simulink model "AirbrakeFlightSim_R2022a"  (R2022a)
settings: Solver=VariableStepAuto  StartTime=0.0  StopTime=18  RelTol=1e-3  AbsTol=1e-6
model workspace (MAT data in the model file):
  test = 1
undefined symbols (not defined in the file or in its folder): accelerometer, atm, gyroscope, model_g_mps2, true_g_mps2, wn, zeta
libraries: simulink x14, simulink_extras x3, aerolibnav x3, matrix_library x2, slpidlib x1
(part 2 of 2)

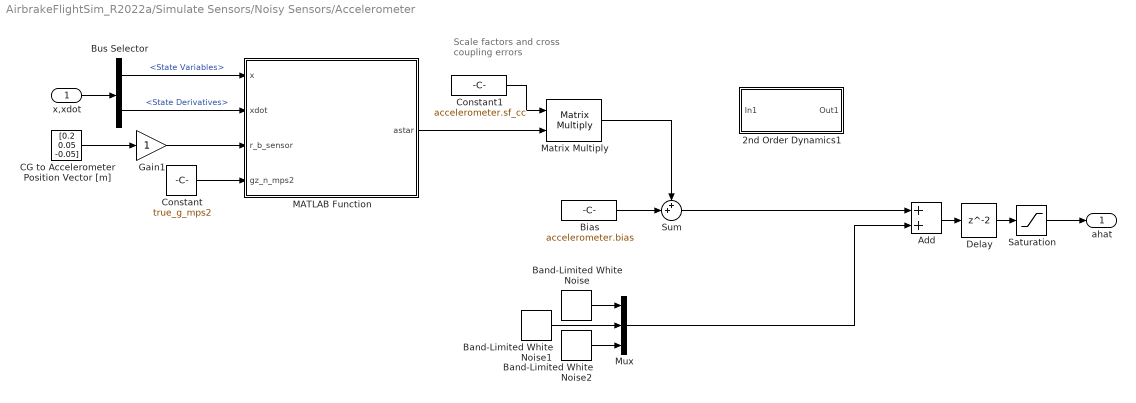
== system AirbrakeFlightSim_R2022a/Simulate Sensors/Noisy Sensors/Accelerometer ==
  note: Scale factors and
      | cross coupling errors
  x,xdot : Inport
  2nd Order Dynamics1 : Subsystem
  Add : Sum
  Band-Limited White Noise : simulink/Sources/Band-Limited White Noise  Cov=[1e-3]  Ts=1/100  seed=[23341]
  Band-Limited White Noise1 : simulink/Sources/Band-Limited White Noise  Cov=[1e-3]  Ts=1/100  seed=[23341]
  Band-Limited White Noise2 : simulink/Sources/Band-Limited White Noise  Cov=[1e-3]  Ts=1/100  seed=[23341]
  Bias : Constant  Value=accelerometer.bias
  Bus Selector : BusSelector  OutputSignals=State Variables,State Derivatives
  CG to Accelerometer Position Vector [m] : Constant  Value=[0.2 0.05 -0.05]
  Constant : Constant  Value=true_g_mps2
  Constant1 : Constant  Value=accelerometer.sf_cc
  Delay : Delay  SampleTime=1/100
  Gain1 : Gain
  MATLAB Function : MATLAB Function  TreatAsAtomicUnit=on
  Matrix Multiply : Product  Multiplication=Matrix(*)
  Mux : Mux  Inputs=3
  Saturation : Saturate  UpperLimit=16*9.81  LowerLimit=-16*9.81
  Sum : Sum  Inputs=++|
  ahat : Outport
  wires:
  Delay/1 -> Saturation/1
  Band-Limited White Noise1/1 -> Mux/2
  Band-Limited White Noise2/1 -> Mux/3
  Band-Limited White Noise/1 -> Mux/1
  Add/1 -> Delay/1
  Saturation/1 -> ahat/1
  x,xdot/1 -> Bus Selector/1
  Bus Selector/1 -> MATLAB Function/1(x)  "<State Variables>"
  Bus Selector/2 -> MATLAB Function/2(xdot)  "<State Derivatives>"
  CG to Accelerometer Position Vector [m]/1 -> Gain1/1
  Constant/1 -> MATLAB Function/4(gz_n_mps2)
  Mux/1 -> Add/2
  Gain1/1 -> MATLAB Function/3(r_b_sensor)
  MATLAB Function/1(astar) -> Matrix Multiply/2
  Constant1/1 -> Matrix Multiply/1
  Sum/1 -> Add/1
  Matrix Multiply/1 -> Sum/1
  Bias/1 -> Sum/2

== system AirbrakeFlightSim_R2022a/Simulate Sensors/Noisy Sensors/Altimeter ==
  x,xdot : Inport
  Add : Sum
  Band-Limited White Noise : simulink/Sources/Band-Limited White Noise  Cov=[0.01]  Ts=1/25  seed=[23341]
  Bus Selector : BusSelector  OutputSignals=State Variables
  Delay1 : Delay  SampleTime=1/25
  Gain : Gain  Gain=-1
  Saturation : Saturate  UpperLimit=20000  LowerLimit=-20000
  Scope : Scope
  Selector : Selector  InputPortWidth=12  IndexOptions=Index vector (dialog)  Indices=[12]  OutputSizes=1
  altitudehat : Outport
  wires:
  Saturation/1 -> altitudehat/1
  Add/1 -> Delay1/1
  Delay1/1 -> Saturation/1
  Selector/1 -> Gain/1  "p_down_m"
  Gain/1 -> Add/1  "altitude"
  x,xdot/1 -> Bus Selector/1
  Bus Selector/1 -> Selector/1  "<State Variables>"
  Band-Limited White Noise/1 -> Add/2

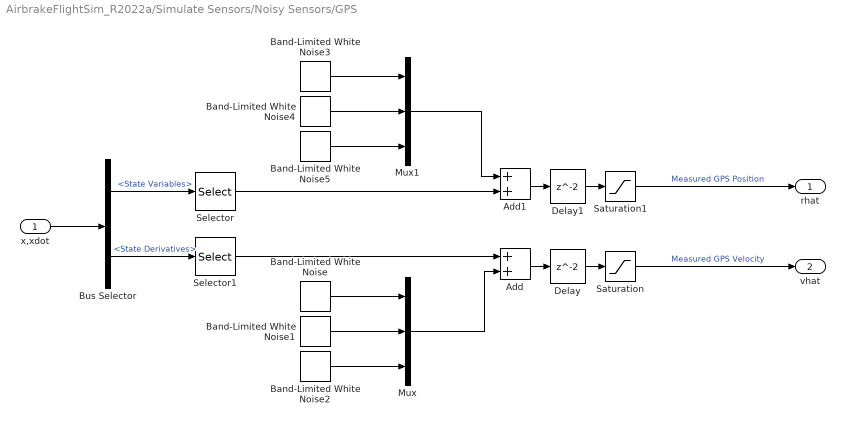
== system AirbrakeFlightSim_R2022a/Simulate Sensors/Noisy Sensors/GPS ==
  x,xdot : Inport
  Add : Sum
  Add1 : Sum
  Band-Limited White Noise{,1..5} (6 alike) : simulink/Sources/Band-Limited White Noise  Cov=[1e-3*pi/180]  Ts=1/100  seed=[23341]
  Bus Selector : BusSelector  OutputSignals=State Variables,State Derivatives
  Delay : Delay  SampleTime=1/100
  Delay1 : Delay  SampleTime=1/100
  Mux : Mux  Inputs=3
  Mux1 : Mux  Inputs=3
  Saturation : Saturate  UpperLimit=500*pi/180  LowerLimit=-500*pi/180
  Saturation1 : Saturate  UpperLimit=500*pi/180  LowerLimit=-500*pi/180
  Selector : Selector  InputPortWidth=12  IndexOptions=Index vector (dialog)  Indices=[10 11 12]  OutputSizes=1
  Selector1 : Selector  InputPortWidth=12  IndexOptions=Index vector (dialog)  Indices=[10 11 12]  OutputSizes=1
  rhat : Outport
  vhat : Outport  Port=2
  wires:
  Delay/1 -> Saturation/1
  Band-Limited White Noise1/1 -> Mux/2
  Band-Limited White Noise2/1 -> Mux/3
  Band-Limited White Noise/1 -> Mux/1
  Add/1 -> Delay/1
  x,xdot/1 -> Bus Selector/1
  Mux/1 -> Add/2
  Bus Selector/1 -> Selector/1  "<State Variables>"
  Bus Selector/2 -> Selector1/1  "<State Derivatives>"
  Band-Limited White Noise5/1 -> Mux1/3
  Band-Limited White Noise4/1 -> Mux1/2
  Band-Limited White Noise3/1 -> Mux1/1
  Selector1/1 -> Add/1
  Add1/1 -> Delay1/1
  Delay1/1 -> Saturation1/1
  Mux1/1 -> Add1/1
  Selector/1 -> Add1/2
  Saturation/1 -> vhat/1  "Measured GPS Velocity"
  Saturation1/1 -> rhat/1  "Measured GPS Position"

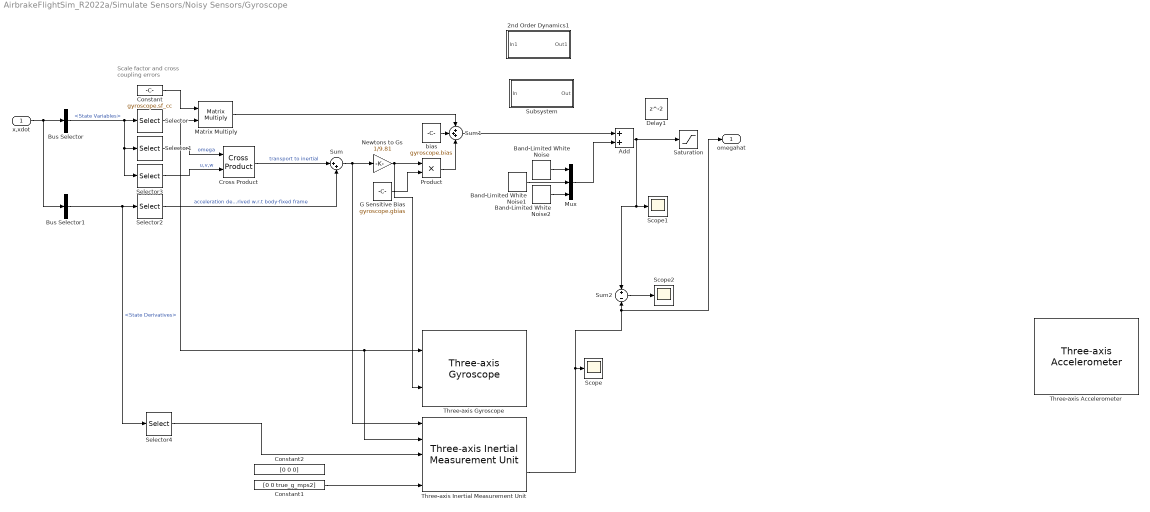
== system AirbrakeFlightSim_R2022a/Simulate Sensors/Noisy Sensors/Gyroscope ==
  note: Scale factor and
      | cross coupling errors
  x,xdot : Inport
  2nd Order Dynamics1 : Subsystem
  Add : Sum
  Band-Limited White Noise : simulink/Sources/Band-Limited White Noise  Cov=[1e-3]  Ts=1/10  seed=23093
  Band-Limited White Noise1 : simulink/Sources/Band-Limited White Noise  Cov=[1e-3]  Ts=1/10  seed=23094
  Band-Limited White Noise2 : simulink/Sources/Band-Limited White Noise  Cov=[1e-3]  Ts=1/10  seed=23095
  Bus Selector : BusSelector  OutputSignals=State Variables
  Bus Selector1 : BusSelector  OutputSignals=State Derivatives
  Constant : Constant  Value=gyroscope.sf_cc
  Constant1 : Constant  Value=[0 0 true_g_mps2]
  Constant2 : Constant  Value=[0 0 0]
  Cross Product : matrix_library/Cross Product
      settings: SourceProductBaseCode=SL
  Delay1 : Delay  SampleTime=1/100
  G Sensitive Bias : Constant  Value=gyroscope.gbias
  Matrix Multiply : Product  Multiplication=Matrix(*)
  Mux : Mux  Inputs=3
  Newtons to Gs : Gain  Gain=1/9.81
  Product : Product
  Saturation : Saturate  UpperLimit=500*pi/180  LowerLimit=-500*pi/180
  Scope : Scope
  Scope1 : Scope
  Scope2 : Scope
  Selector : Selector  InputPortWidth=12  IndexOptions=Index vector (dialog)  Indices=[4 5 6]  OutputSizes=1
  Selector1 : Selector  InputPortWidth=12  IndexOptions=Index vector (dialog)  Indices=[4 5 6]  OutputSizes=1
  Selector2 : Selector  InputPortWidth=12  IndexOptions=Index vector (dialog)  Indices=[1 2 3]  OutputSizes=1
  Selector3 : Selector  InputPortWidth=12  IndexOptions=Index vector (dialog)  Indices=[1 2 3]  OutputSizes=1
  Selector4 : Selector  InputPortWidth=12  IndexOptions=Index vector (dialog)  Indices=[4 5 6]  OutputSizes=1
  Subsystem : Subsystem
  Sum : Sum  Inputs=|++
  Sum1 : Sum  Inputs=+++
  Sum2 : Sum  Inputs=+|-
  Three-axis Accelerometer : aerolibnav/Three-axis Accelerometer  units=Metric (MKS)  acc=[0 0 0]  gtype=on  dtype_a=on  w_a=190  z_a=0.707  a_sf_cc=[1 0 0; 0 1 0; 0 0 1]  a_bias=[0 0 0]  a_Ts=0  a_rand=on  a_seeds=[23093 23094 23095]  a_pow=[0.001 0.001 0.001]  a_sat="[-inf  -inf  -inf  inf inf inf]"
      settings: SourceProductBaseCode=AE
  Three-axis Gyroscope : aerolibnav/Three-axis Gyroscope  dtype_g=on  w_g=wn  z_g=zeta  g_sf_cc=gyroscope.sf_cc  g_bias=gyroscope.bias  g_sen=gyroscope.gbias  g_Ts=1/100  g_rand=on  g_seeds=[23093 23094 23095]  g_pow=[0.001 0.001 0.001]  g_sat="[-inf  -inf  -inf  inf inf inf]"
      settings: SourceProductBaseCode=AE
  Three-axis Inertial Measurement Unit : aerolibnav/Three-axis Inertial Measurement Unit  units=Metric (MKS)  imu=[0 0 0]  i_Ts=0  dtype_a=off  w_a=wn  z_a=zeta  a_sf_cc=[1 0 0; 0 1 0; 0 0 1]  a_bias=[0 0 0]  a_sat="[-inf  -inf  -inf  inf inf inf]"  dtype_g=off  w_g=wn  z_g=zeta  g_sf_cc=[1 0 0; 0 1 0; 0 0 1]  g_bias=[0 0 0]  g_sens=[0 0 0]  g_sat="[-inf  -inf  -inf  inf inf inf]"  i_rand=on  i_seeds=[23093 23094 23095 23093 23094 23095]  i_pow=[0.001 0.001 0.001 0.001 0.001 0.001]
  bias : Constant  Value=gyroscope.bias
  omegahat : Outport
  wires:
  Add/1 -> Saturation/1, Sum2/1, Scope1/1
  Band-Limited White Noise1/1 -> Mux/2
  Band-Limited White Noise2/1 -> Mux/3
  Band-Limited White Noise/1 -> Mux/1
  x,xdot/1 -> Bus Selector1/1, Bus Selector/1
  Bus Selector/1 -> Selector/1, Selector3/1, Selector1/1  "<State Variables>"
  Mux/1 -> Add/2
  Selector/1 -> Three-axis Gyroscope/1, Three-axis Inertial Measurement Unit/2, Matrix Multiply/2
  Constant/1 -> Matrix Multiply/1
  Bus Selector1/1 -> Selector4/1, Selector2/1  "<State Derivatives>"
  Selector3/1 -> Cross Product/2  "u,v,w"
  Selector1/1 -> Cross Product/1  "omega"
  Cross Product/1 -> Sum/1  "transport to inertial"
  Selector2/1 -> Sum/2  "acceleration derived w.r.t body-fixed frame"
  Sum/1 -> Newtons to Gs/1, Three-axis Inertial Measurement Unit/1
  Newtons to Gs/1 -> Product/1, Three-axis Gyroscope/2
  G Sensitive Bias/1 -> Product/2
  Product/1 -> Sum1/3
  Matrix Multiply/1 -> Sum1/1
  bias/1 -> Sum1/2
  Three-axis Inertial Measurement Unit/2 -> omegahat/1, Sum2/2, Scope/1
  Sum2/1 -> Scope2/1
  Selector4/1 -> Three-axis Inertial Measurement Unit/3
  Constant1/1 -> Three-axis Inertial Measurement Unit/5
  Sum1/1 -> Add/1

== system AirbrakeFlightSim_R2022a/Simulate Sensors/Noisy Sensors/Magnetometer ==
  x,xdot : Inport
  Add : Sum
  Band-Limited White Noise : simulink/Sources/Band-Limited White Noise  Cov=[0.01]  Ts=1/25  seed=[23341]
  Bus Selector : BusSelector  OutputSignals=State Variables
  Delay1 : Delay  SampleTime=1/25
  Saturation : Saturate  UpperLimit=20000  LowerLimit=-20000
  Selector : Selector  InputPortWidth=12  IndexOptions=Index vector (dialog)  Indices=[9]  OutputSizes=1
  headinghat : Outport
  wires:
  Saturation/1 -> headinghat/1
  Add/1 -> Delay1/1
  Delay1/1 -> Saturation/1
  Selector/1 -> Add/1  "yaw"
  x,xdot/1 -> Bus Selector/1
  Bus Selector/1 -> Selector/1  "<State Variables>"
  Band-Limited White Noise/1 -> Add/2

== system AirbrakeFlightSim_R2022a/Simulate True Dynamics 6DOF/Compute Aerodynamic Forces/Angle of Attack ==
  In1 : Inport
  Atan2 : Trigonometry  Operator=atan2
  Demux : Demux  Outputs=3
  alpha : Outport
  wires:
  In1/1 -> Demux/1
  Atan2/1 -> alpha/1
  Demux/3 -> Atan2/1
  Demux/1 -> Atan2/2

== system AirbrakeFlightSim_R2022a/Simulate True Dynamics 6DOF/Compute Aerodynamic Forces/Angle of Sideslip ==
  v : Inport
  V : Inport  Port=2
  Abs : Abs  SaturateOnIntegerOverflow=off
  Asin : Trigonometry  Operator=asin
  Constant : Constant  Value=0
  Divide : Product  Inputs=*/
  Selector : Selector  InputPortWidth=3  IndexOptions=Index vector (dialog)  Indices=[2]  OutputSizes=1
  Switch : Switch  Criteria=u2 > Threshold  SaturateOnIntegerOverflow=off  InputSameDT=off
  beta : Outport
  wires:
  V/1 -> Divide/2
  Divide/1 -> Asin/1
  Asin/1 -> Switch/1, Abs/1
  Switch/1 -> beta/1
  Abs/1 -> Switch/2
  Constant/1 -> Switch/3
  v/1 -> Selector/1
  Selector/1 -> Divide/1

== system AirbrakeFlightSim_R2022a/Simulate True Dynamics 6DOF/Compute Aerodynamic Forces/Dynamic Pressure ==
  V : Inport
  rho : Inport  Port=2
  Constant : Constant  Value=0.5
  Product : Product  Inputs=4
  qbar : Outport
  wires:
  V/1 -> Product/3, Product/2
  rho/1 -> Product/4
  Constant/1 -> Product/1
  Product/1 -> qbar/1

== system AirbrakeFlightSim_R2022a/Simulate True Dynamics 6DOF/Compute Aerodynamic Forces/Mach Number ==
  V : Inport
  c : Inport  Port=2
  Divide : Product  Inputs=*/
  M : Outport
  wires:
  V/1 -> Divide/1
  c/1 -> Divide/2
  Divide/1 -> M/1

== system AirbrakeFlightSim_R2022a/Simulate True Dynamics 6DOF/Compute Aerodynamic Forces/Speed of Sound ==
  Temperature : Inport
  Ratio of specific heats : Gain  Gain=1.4
  Specific gas constant : Gain  Gain=287.05
  Sqrt : Sqrt
  c : Outport
  wires:
  Temperature/1 -> Ratio of specific heats/1
  Ratio of specific heats/1 -> Specific gas constant/1
  Specific gas constant/1 -> Sqrt/1
  Sqrt/1 -> c/1

== system AirbrakeFlightSim_R2022a/Simulate True Dynamics 6DOF/Interpolate Thrust & Mass/Check Motor Burnout ==
  In1 : Inport
  Bus Selector : BusSelector  OutputSignals=Vehicle Properties.Motor Time Breakpoints,Simulation Time
  Gain : Gain  Gain=-1
  checkMotorBurnout : Subsystem
  tag scope: Time_Since_Burnout=global
  wires:
  checkMotorBurnout/1(Time Since Burnout) -> [Time_Since_Burnout]
  In1/1 -> Bus Selector/1
  Bus Selector/1 -> Gain/1  "<Motor Time Breakpoints>"
  Bus Selector/2 -> checkMotorBurnout/2(In2)  "<Simulation Time>"
  Gain/1 -> checkMotorBurnout/1(In1)

== system AirbrakeFlightSim_R2022a/Simulate True Dynamics 6DOF/Interpolate Thrust & Mass/Inertia (UNFINISHED) ==
  In1 : Inport
  Bus Selector : BusSelector  OutputSignals=Vehicle Properties.Vehicle Inertia [kg-m2]
  Out1 : Outport
  wires:
  In1/1 -> Bus Selector/1
  Bus Selector/1 -> Out1/1  "<Vehicle Inertia [kg-m2]>"

== system AirbrakeFlightSim_R2022a/Simulate True Dynamics 6DOF/Interpolate Thrust & Mass/Interpolate Mass ==
  1 : Inport
  Add : Sum
  Bus Selector : BusSelector  OutputSignals=Vehicle Properties.Vehicle Mass [kg],Simulation Time,Vehicle Properties.Motor Mass Breakpoints,Vehicle Properties.Motor Time Breakpoints
  Mass Curve : Lookup_n-D  NumberOfTableDimensions=1  BreakpointsForDimension1Source=Input port  BreakpointsForDimension1=|  TableSource=Input port  Table=|  ExtrapMethod=Clip  UseLastTableValue=on  InternalRulePriority=Speed  RndMeth=Simplest
      BreakpointsForDimension1=|
      | [   2.0000e-02
      |    4.0000e-02
      |    5.5000e-02
      |    7.3000e-02
      |    1.5600e-01
      |    3.9700e-01
      |    6.9100e-01
      |    9.8200e-01
      |    1.4100e+00
      |    1.6960e+00
      |    1.9350e+00
      |    2.0600e+00
      |    2.1030e+00
      |    2.1160e+00
      |    2.1330e+00
      |    2.1630e+00
      |    2.2140e+00
      |    2.2440e+00
      |    2.2960e+00
      |    2.3090e+00]
      Table=|
      | [4.8137e+01
      |    2.1073e+03
      |    2.2892e+03
      |    2.1501e+03
      |    2.1020e+03
      |    2.1501e+03
      |    2.1555e+03
      |    2.1180e+03
      |    2.0004e+03
      |    1.8987e+03
      |    1.8399e+03
      |    1.8185e+03
      |    1.6527e+03
      |    1.3746e+03
      |    9.3600e+02
      |    5.3486e+02
      |    2.4069e+02
      |    1.1232e+02
      |    5.3490e+00
      |             0]
      settings: InputPortMap=u0,p221,p5
  Mass : Outport
  wires:
  Mass Curve/1 -> Add/2
  Add/1 -> Mass/1
  1/1 -> Bus Selector/1
  Bus Selector/2 -> Mass Curve/1  "<Simulation Time>"
  Bus Selector/3 -> Mass Curve/2  "<Motor Mass Breakpoints>"
  Bus Selector/4 -> Mass Curve/3  "<Motor Time Breakpoints>"
  Bus Selector/1 -> Add/1  "<Vehicle Mass [kg]>"

== system AirbrakeFlightSim_R2022a/Simulate True Dynamics 6DOF/Interpolate Thrust & Mass/Interpolate Thrust ==
  In1 : Inport
  Bus Selector : BusSelector  OutputSignals=Motor Thrust Breakpoints,Motor Time Breakpoints
  Bus Selector1 : BusSelector  OutputSignals=Simulation Time,Vehicle Properties
  "Thrust Curve " : Lookup_n-D  NumberOfTableDimensions=1  BreakpointsForDimension1Source=Input port  BreakpointsForDimension1=|  TableSource=Input port  Table=|  ExtrapMethod=Clip  InternalRulePriority=Speed  RndMeth=Simplest
      BreakpointsForDimension1=|
      | [   2.0000e-02
      |    4.0000e-02
      |    5.5000e-02
      |    7.3000e-02
      |    1.5600e-01
      |    3.9700e-01
      |    6.9100e-01
      |    9.8200e-01
      |    1.4100e+00
      |    1.6960e+00
      |    1.9350e+00
      |    2.0600e+00
      |    2.1030e+00
      |    2.1160e+00
      |    2.1330e+00
      |    2.1630e+00
      |    2.2140e+00
      |    2.2440e+00
      |    2.2960e+00
      |    2.3090e+00]
      Table=|
      | [4.8137e+01
      |    2.1073e+03
      |    2.2892e+03
      |    2.1501e+03
      |    2.1020e+03
      |    2.1501e+03
      |    2.1555e+03
      |    2.1180e+03
      |    2.0004e+03
      |    1.8987e+03
      |    1.8399e+03
      |    1.8185e+03
      |    1.6527e+03
      |    1.3746e+03
      |    9.3600e+02
      |    5.3486e+02
      |    2.4069e+02
      |    1.1232e+02
      |    5.3490e+00
      |             0]
      settings: InputPortMap=u0,p221,p5
  Out1 : Outport
  wires:
  "Thrust Curve "/1 -> Out1/1
  Bus Selector/2 -> "Thrust Curve "/3  "<Motor Time Breakpoints>"
  Bus Selector/1 -> "Thrust Curve "/2  "<Motor Thrust Breakpoints>"
  Bus Selector1/1 -> "Thrust Curve "/1  "<Simulation Time>"
  In1/1 -> Bus Selector1/1
  Bus Selector1/2 -> Bus Selector/1  "<Vehicle Properties>"

== system AirbrakeFlightSim_R2022a/Simulate Sensors/Noisy Sensors/Accelerometer/2nd Order Dynamics1 ==
  In1 : Inport
  Gain : Gain  Gain=wn*wn
  Gain1 : Gain  Gain=2*zeta*wn
  "Integrator, Second-Order" : SecondOrderIntegrator
  Sum : Sum  Inputs=|++
  Sum1 : Sum  Inputs=|++
  Out1 : Outport
  wires:
  In1/1 -> Sum/1
  Sum/1 -> Gain/1
  Gain/1 -> Sum1/1
  Sum1/1 -> "Integrator, Second-Order"/1
  "Integrator, Second-Order"/1 -> Sum/2, Out1/1
  "Integrator, Second-Order"/2 -> Gain1/1
  Gain1/1 -> Sum1/2

== system AirbrakeFlightSim_R2022a/Simulate Sensors/Noisy Sensors/Gyroscope/2nd Order Dynamics1 ==
  In1 : Inport
  Gain : Gain  Gain=wn*wn
  Gain1 : Gain  Gain=2*zeta*wn
  "Integrator, Second-Order" : SecondOrderIntegrator
  Sum : Sum  Inputs=|+-
  Sum1 : Sum  Inputs=|+-
  Out1 : Outport
  wires:
  In1/1 -> Sum/1
  Sum/1 -> Gain/1
  Gain/1 -> Sum1/1
  Sum1/1 -> "Integrator, Second-Order"/1
  "Integrator, Second-Order"/1 -> Sum/2, Out1/1
  "Integrator, Second-Order"/2 -> Gain1/1
  Gain1/1 -> Sum1/2

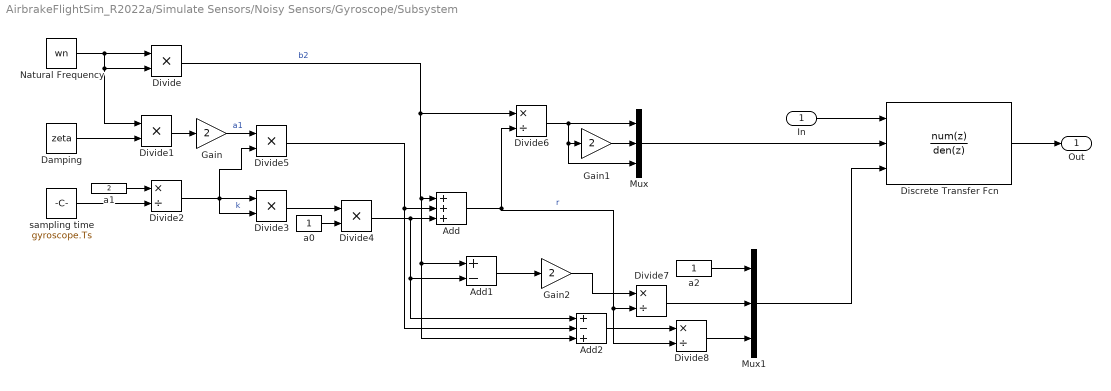
== system AirbrakeFlightSim_R2022a/Simulate Sensors/Noisy Sensors/Gyroscope/Subsystem ==
  In : Inport
  Add : Sum  Inputs=+++
  Add1 : Sum  Inputs=+-
  Add2 : Sum  Inputs=+-+
  Damping : Constant  Value=zeta
  Discrete Transfer Fcn : DiscreteTransferFcn  NumeratorSource=Input port  DenominatorSource=Input port  SampleTime=gyroscope.Ts  a0EqualsOne=on
      settings: InputPortMap=u0,p1,p3
  Divide{,1,3..5} (5 alike) : Product  Inputs=**
  Divide{2,6..8} (4 alike) : Product  Inputs=*/
  Gain : Gain  Gain=2
  Gain1 : Gain  Gain=2
  Gain2 : Gain  Gain=2
  Mux : Mux  Inputs=3
  Mux1 : Mux  Inputs=3
  Natural Frequency : Constant  Value=wn
  a0 : Constant
  a1 : Constant  Value=2
  a2 : Constant
  sampling time : Constant  Value=gyroscope.Ts
  Out : Outport  VectorParamsAs1DForOutWhenUnconnected=off
  wires:
  Divide1/1 -> Gain/1
  Divide8/1 -> Mux1/3
  Divide7/1 -> Mux1/2
  Divide2/1 -> Divide5/2, Divide3/2, Divide3/1  "k"
  Add/1 -> Divide8/2, Divide7/2, Divide6/2  "r"
  In/1 -> Discrete Transfer Fcn/1
  Gain/1 -> Divide5/1  "a1"
  Mux1/1 -> Discrete Transfer Fcn/3
  Add1/1 -> Gain2/1
  Mux/1 -> Discrete Transfer Fcn/2
  Gain1/1 -> Mux/2
  Divide5/1 -> Add2/2, Add/2
  Gain2/1 -> Divide7/1
  Add2/1 -> Divide8/1
  sampling time/1 -> Divide2/2
  a1/1 -> Divide2/1
  Divide3/1 -> Divide4/1
  Divide4/1 -> Add2/1, Add1/2, Add/3
  a2/1 -> Mux1/1
  Divide/1 -> Divide6/1, Add2/3, Add1/1, Add/1  "b2"
  a0/1 -> Divide4/2
  Damping/1 -> Divide1/2
  Discrete Transfer Fcn/1 -> Out/1
  Natural Frequency/1 -> Divide/1, Divide/2, Divide1/1
  Divide6/1 -> Mux/3, Gain1/1, Mux/1

== system AirbrakeFlightSim_R2022a/Simulate True Dynamics 6DOF/Interpolate Thrust & Mass/Check Motor Burnout/checkMotorBurnout ==
  In1 : Inport
  In2 : Inport  Port=2
  Add : Sum
  Selector : Selector  InputPortWidth=20  IndexOptions=Index vector (dialog)  Indices=[20]  OutputSizes=1
  Time Since Burnout : Outport
  wires:
  Selector/1 -> Add/1
  Add/1 -> Time Since Burnout/1
  In2/1 -> Add/2
  In1/1 -> Selector/1

== matlab function AirbrakeFlightSim_R2022a/Simulate True Dynamics 6DOF/Compute Aerodynamic Forces/MATLAB Function ==
  data: drag_characteristics input; fins input; velocity_vec input; D output; alpha_rad input; beta_rad input; qbar_kgpms2 input; mach input; Y output; L output
function [D,Y,L] = compute_aerodynamic_forces(drag_characteristics,fins, velocity_vec, alpha_rad,beta_rad,qbar_kgpms2, mach)
% aero_w_N = rocketAeroModel(alpha_rad, beta_rad, qbar_kgpms2, vehicle)
% 
% Computes the aerodynamic force vector of launch vehicle with fins placed
% symmetrically about the longitudinal axis. The body-fixed frame must
% have the y-axis along any fin.
% 
% Inputs:
%   drag_characteristics - vehicle CD*S   
%
%   fins - vector containing vehicle parameters
%       fins.num_fins - number of fins
%       fins.CL_alpha - slope of the lift coeff vs angle of attack curve
%       fins.planform_area - exposed planform area of fin
%
%   velocity_vec - 3x1 vector containing u,v,w body-fixed inertial velocities
%
%   alpha_rad - vehicle angle of attack in radians
%
%   beta_rad - vehicle angle of sideslip in radians
%
%   qbar_kgpms2 - vehicle dynamic pressure in Newtons per meter squared
%
%   mach - mach number
%
% Outputs:
%   aero_B_N - aerodynamic force vector resolved in Body-Fixed coordinates
%   and expressed in Newtons.
%       3 x 1 vector

%% Old Attempt
% % Extract vehicle properties
% CL_alpha = vehicle.fins.CL_alpha;
% CD = vehicle.cd;
% vehicle_area = vehicle.area;
% 
% % Compute drag (fixed Cd does not vary with AoA)
% D = CD*qbar_kgpms2*vehicle_area;
% 
% % Compute lift coeff
% CL = CL_alpha * alpha_rad;
% L = CL*qbar_kgpms2*vehicle_area;
% 
% aero_w_N = [D 0 L];

%% New attempt

% Define vehicle parameters
C_N_alpha_fins = fins(1);
fin_area = fins(2);
num_fins = fins(3);
C_N_alpha_nosecone = 2;


% Initialize aerodynamic force vector resolved in wind axes
aero_w_N = [0 0 0]';

% Fins
for ii = 0:num_fins-1
    
    % Fin position along body diameter
    psi = (2*pi/num_fins)*ii;

    % angle of attack relative to i'th fin
    alpha_i = alpha_rad*cos(psi) - beta_rad*sin(psi);

    % Magnitude of normal force from i'th fin
    N = qbar_kgpms2 * fin_area * C_N_alpha_fins * alpha_i;

    % Direction of normal force
    n_hat = [0 -sin(psi) cos(psi)]';

    % Normal force vector for i'th fin
    F_i = N*n_hat;
    
    % Add to total aerodynamic force
    aero_w_N = aero_w_N + F_i;
end

% Nose cone (try and figure out why this doesnt effect pitch at apogee?)
alpha_eff = acos(velocity_vec(1)/norm(velocity_vec));
if isnan(alpha_eff)
    alpha_eff = 0;
end
N = qbar_kgpms2 * fin_area * C_N_alpha_nosecone * alpha_eff;
F_nosecone = N*[0 0 1]';
aero_w_N = aero_w_N + F_nosecone;

D = qbar_kgpms2*drag_characteristics;
aero_w_N = aero_w_N + [D 0 0]';

% Extract components
aero_w_N = -aero_w_N;
D = aero_w_N(1);
Y = aero_w_N(2);
L = aero_w_N(3);

== matlab function AirbrakeFlightSim_R2022a/Simulate True Dynamics 6DOF/Net Force/MATLAB Function ==
  data: alpha_rad input size=1; beta_rad input size=1; aero_w_N input size=3; aero_b_N output size=3
function aero_b_N = convert_aero_w2b(alpha_rad,beta_rad,aero_w_N)
% Transforms aerodynamic forces resolved in wind axes to aerodynamic forces
% resolved in body-fixed axes
% 
% Inputs:
%   alpha_rad   :   angle of attack [rad]
%   beta_rad    :   angle of sideslip [rad]
%   aero_w_N    :   aerodynamic force vector resolved in wind axes [N]
%
% Outputs:
%   aero_b_N    :   aerodynamic force vector resolved in body axes [N]
%

% Store trig ops
s_alpha = sin(alpha_rad);
c_alpha = cos(alpha_rad);
s_beta = sin(beta_rad);
c_beta = cos(beta_rad);

% wind to body DCM
C_w2b_11 =  c_alpha*c_beta;
C_w2b_12 = -c_alpha*s_beta;
C_w2b_13 = -s_alpha;
C_w2b_21 =  s_beta;
C_w2b_22 =  c_beta;
C_w2b_23 =  0;
C_w2b_31 =  s_alpha*c_beta;
C_w2b_32 = -s_alpha*s_beta;
C_w2b_33 =  c_alpha;

% Extract aerodynamic force components in wind axes
xaero_w_N = aero_w_N(1);
yaero_w_N = aero_w_N(2);
zaero_w_N = aero_w_N(3);

% Rotate aerodynamic forces to body axes
xaero_b_N = C_w2b_11*xaero_w_N + C_w2b_12*yaero_w_N + C_w2b_13*zaero_w_N;
yaero_b_N = C_w2b_21*xaero_w_N + C_w2b_22*yaero_w_N + C_w2b_23*zaero_w_N;
zaero_b_N = C_w2b_31*xaero_w_N + C_w2b_32*yaero_w_N + C_w2b_33*zaero_w_N;

% Compile vector components
aero_b_N = [xaero_b_N yaero_b_N zaero_b_N]';

== matlab function AirbrakeFlightSim_R2022a/Simulate True Dynamics 6DOF/Compute State Variables/MATLAB Function ==
  data: x input; xdot output; Fvec_b_N input; Mvec_b_N input; J_tensor_b_kgm2 input; m_kg input; gvec_b_mps2 input
function xdot = flat_earth_eom(x, Fvec_b_N, Mvec_b_N, J_tensor_b_kgm2, m_kg, gvec_b_mps2)

%% Parse Inputs
% Extract state variables
u_b_mps = x(1);  % Body-fixed velocities along x,y,z
v_b_mps = x(2);
w_b_mps = x(3);
p_b_rps = x(4);  % Body-fixed angular velocities along x,y,z
q_b_rps = x(5);
r_b_rps = x(6);
phi_rad = x(7);  % Euler-angles roll,pitch,yaw
theta_rad = x(8);
psi_rad = x(9);
p1_n_m = x(10);  % Inertial position north,east,down
p2_n_m = x(11);
p3_n_m = x(12);

% Store trigonometric operations
s_phi = sin(phi_rad);
c_phi = cos(phi_rad);
s_theta = sin(theta_rad);
c_theta = cos(theta_rad);
t_theta = tan(theta_rad);
s_psi = sin(psi_rad);
c_psi = cos(psi_rad);

% Inertia
Jxx_b_kgm2 = J_tensor_b_kgm2(1,1);
Jyy_b_kgm2 = J_tensor_b_kgm2(2,2);
Jzz_b_kgm2 = J_tensor_b_kgm2(3,3);
Jxz_b_kgm2 = J_tensor_b_kgm2(1,3);

% Compute Body-fixed to NED DCM
C_b2n_11 =  c_theta*c_psi;
C_b2n_12 = -c_phi*s_psi + s_phi*s_theta*c_psi;
C_b2n_13 =  s_phi*s_psi + c_phi*s_theta*c_psi;
C_b2n_21 =  c_theta*s_psi;
C_b2n_22 =  c_phi*c_psi + s_phi*s_theta*s_psi;
C_b2n_23 = -s_phi*c_psi + c_phi*s_theta*s_psi;
C_b2n_31 = -s_theta;
C_b2n_32 =  s_phi*c_theta;
C_b2n_33 =  c_phi*c_theta;

% Forces
Fx_b_N = Fvec_b_N(1);
Fy_b_N = Fvec_b_N(2);
Fz_b_N = Fvec_b_N(3);

% Moments
l_b_Nm = Mvec_b_N(1);
m_b_Nm = Mvec_b_N(2);
n_b_Nm = Mvec_b_N(3);

% Gravitational Acceleration
gx_b_mps2 = gvec_b_mps2(1);
gy_b_mps2 = gvec_b_mps2(2);
gz_b_mps2 = gvec_b_mps2(3);

%% State derivatives
xdot = zeros(12,1);

% Denominator in roll and yaw rate equations (might change for rocket)
Den = Jxx_b_kgm2 * Jzz_b_kgm2  - Jxz_b_kgm2^2;

% position rates
xdot(1) = 1/m_kg * Fx_b_N + gx_b_mps2 - w_b_mps*q_b_rps + v_b_mps*r_b_rps;  % vx
xdot(2) = 1/m_kg * Fy_b_N + gy_b_mps2 - u_b_mps*r_b_rps + w_b_mps*p_b_rps;  % vy
xdot(3) = 1/m_kg * Fz_b_N + gz_b_mps2 - v_b_mps*p_b_rps + u_b_mps*q_b_rps;  % vz

% angular rates
xdot(4) = ( Jxz_b_kgm2*(Jxx_b_kgm2 - Jyy_b_kgm2 + Jzz_b_kgm2)*p_b_rps*q_b_rps ...
            - (Jzz_b_kgm2*(Jzz_b_kgm2-Jyy_b_kgm2)+Jxz_b_kgm2^2)*q_b_rps*r_b_rps ...
            + Jzz_b_kgm2*l_b_Nm + Jxz_b_kgm2*n_b_Nm ) / Den;                % roll rate
xdot(5) = ( (Jzz_b_kgm2 - Jxx_b_kgm2)*r_b_rps*p_b_rps - Jxz_b_kgm2*(p_b_rps^2-r_b_rps^2) + m_b_Nm ) / Jyy_b_kgm2;  % pitch rate
xdot(6) = ( -Jxz_b_kgm2*(Jxx_b_kgm2 - Jyy_b_kgm2 + Jzz_b_kgm2)*q_b_rps*r_b_rps...
            + (Jxx_b_kgm2*(Jxx_b_kgm2 - Jyy_b_kgm2) + Jxz_b_kgm2^2)*p_b_rps*q_b_rps ...
            + Jxz_b_kgm2*l_b_Nm+Jxx_b_kgm2*n_b_Nm ) / Den;  % yaw rate
% euler kinematics
xdot(7) = p_b_rps + s_phi*t_theta*q_b_rps + c_phi*t_theta*r_b_rps;
xdot(8) = c_phi*q_b_rps - s_phi*r_b_rps;
xdot(9) = s_phi/c_theta*q_b_rps + c_phi/c_theta*r_b_rps;
% navigation equations
xdot(10) = C_b2n_11*u_b_mps + C_b2n_12*v_b_mps + C_b2n_13*w_b_mps;  % x-vel resolved in NED
xdot(11) = C_b2n_21*u_b_mps + C_b2n_22*v_b_mps + C_b2n_23*w_b_mps;  % y-vel in NED
xdot(12) = C_b2n_31*u_b_mps + C_b2n_32*v_b_mps + C_b2n_33*w_b_mps;  % z-vel in NED

== matlab function AirbrakeFlightSim_R2022a/Predict Apogee/PREDICT APOGEE ==
  data: dragConstant input; velocity input; position input; y output
function y = fcn(dragConstant, velocity, position)
    y = 0;
    
    px = sqrt(position(1)^2 + position(2)^2);
    vx = sqrt(velocity(1)^2 + velocity(2)^2);

    py = -position(3);
    vy = -velocity(3);

    ic = [px vx py vy];
    y = mainSIMULINK(dragConstant, ic);
end

== matlab function AirbrakeFlightSim_R2022a/Simulate Sensors/Ideal Sensors/MATLAB Function ==
  data: astar output; x input; xdot input; r_b_sensor input; gz_n_mps2 input
function astar = simulateIdealAccelerometer(x,xdot,r_b_sensor,gz_n_mps2)
% function astar = simulateAccelerometer(x,xdot,r_sensor)
% Generates idealized accelerometer readings
%
% Inputs:
%   x - state vector [u v w p q r phi theta psi p_N p_E p_D]'
%   xdot - state derivative
%   r_sensor - position vector of accelerometer w.r.t. vehicle CM
%
% Outputs:
%   astar = idealized accelerometer readings (no bias, drift, noise).
%

% Extract state variables
phi_rad = x(7);  % Euler-angles roll,pitch
theta_rad = x(8);

% Store trigonometric operations
s_phi = sin(phi_rad);
c_phi = cos(phi_rad);
s_theta = sin(theta_rad);
c_theta = cos(theta_rad);

% Define NED to body-fixed rotation 
C_n2b_13 = -s_theta;
C_n2b_23 = s_phi*c_theta;
C_n2b_33 = c_phi*c_theta;

% Resolve gravity in body-fixed
gx_b_mps2 = C_n2b_13*gz_n_mps2;
gy_b_mps2 = C_n2b_23*gz_n_mps2;
gz_b_mps2 = C_n2b_33*gz_n_mps2;
g_b_mps2 = [gx_b_mps2 gy_b_mps2 gz_b_mps2]';

% Extract vectors
vvec = [x(1) x(2) x(3)]';
vvecdot = [xdot(1) xdot(2) xdot(3)]';
omega = [x(4) x(5) x(6)]';
omegadot = [xdot(4) xdot(5) xdot(6)]';

% Compute idealized accelerometer readings
astar = vvecdot + cross(omega,vvec) + cross(omegadot,r_b_sensor)...
    + cross(omega, cross(omega, r_b_sensor)) - g_b_mps2;

== matlab function AirbrakeFlightSim_R2022a/Navigation/Dead Reckoning/MATLAB Function ==
  data: Theta input; Thetadot output; omega_rps input
function Thetadot = compute_euler_rates(Theta, omega_rps)
% function dTheta = compute_euler_rates(Theta, omega_rad)
% compute_euler_rates computes the time derivative of the euler angles
% roll, pitch, and yaw as a function of the euler angles and the body-fixed
% angular rates.
%
% Inputs:
%   Theta - 3x1 vector containing roll, pitch, yaw
%   omega_rad - 3x1 vector containing p,q,r
%
% Outputs:
%   Thetadot - 3x1 vector containing time derivatives of roll, pitch, yaw
%

% Extract Euler Angles
phi_rad = Theta(1);
theta_rad = Theta(2);

% Compute transformation from p,q,r to euler angle rates
T = [1, sin(phi_rad)*tan(theta_rad), cos(phi_rad)*tan(theta_rad);
        0, cos(phi_rad), -sin(phi_rad);
        0, sin(phi_rad)/cos(theta_rad), cos(phi_rad)/cos(theta_rad)];

% Transform p,q,r
Thetadot = T * omega_rps;

end

== matlab function AirbrakeFlightSim_R2022a/Navigation/Dead Reckoning/MATLAB Function1 ==
  data: gz_n_mps2 input; a_meas input; Theta input; avec_n_mps2 output
function avec_n_mps2 = inertial_acceleration(gz_n_mps2, a_meas, Theta)
%

% Extract euler angles
phi_rad = Theta(1);
theta_rad = Theta(2);
psi_rad = Theta(3);

% Store trigonometric operations
s_phi = sin(phi_rad);
c_phi = cos(phi_rad);
s_theta = sin(theta_rad);
c_theta = cos(theta_rad);
s_psi = sin(psi_rad);
c_psi = cos(psi_rad);

% Compute Body-fixed to NED DCM
C_b2n_11 =  c_theta*c_psi;
C_b2n_12 = -c_phi*s_psi + s_phi*s_theta*c_psi;
C_b2n_13 =  s_phi*s_psi + c_phi*s_theta*c_psi;
C_b2n_21 =  c_theta*s_psi;
C_b2n_22 =  c_phi*c_psi + s_phi*s_theta*s_psi;
C_b2n_23 = -s_phi*c_psi + c_phi*s_theta*s_psi;
C_b2n_31 = -s_theta;
C_b2n_32 =  s_phi*c_theta;
C_b2n_33 =  c_phi*c_theta;

% Extract measured accel components
a_meas_x = a_meas(1);
a_meas_y = a_meas(2);
a_meas_z = a_meas(3);

% Compute inertial acceleration
ax = C_b2n_11*a_meas_x + C_b2n_12*a_meas_y + C_b2n_13*a_meas_z;
ay = C_b2n_21*a_meas_x + C_b2n_22*a_meas_y + C_b2n_23*a_meas_z;
az = C_b2n_31*a_meas_x + C_b2n_32*a_meas_y + C_b2n_33*a_meas_z + gz_n_mps2;
avec_n_mps2 = [ax ay az]';

== matlab function AirbrakeFlightSim_R2022a/Navigation/Dead Reckoning/MATLAB Function2 ==
  data: vec_n input; vec_b output; Theta input
function vec_b = rotateN2B(vec_n, Theta)
% function vec_b_mps = rotateN2B(vec_n_mps, Theta)
% Rotates a vector resolved in navigation coordinates to body-fixed coordinates
%
% Inputs:
%   vec_n - 3 x 1 vector resolved in navigation coordinates
%   Theta - 3 x 1 vector containing Euler angles phi, theta, psi in radians
%
% Outputs:
%   vec_b - transformed 3 x 1 vector resolved in body-fixed coordinates
%

% Extract Euler Angles
phi_rad = Theta(1);
theta_rad = Theta(2);
psi_rad = Theta(3);

% Extract NED velocity components
u_n_mps = vec_n(1);
v_n_mps = vec_n(2);
w_n_mps = vec_n(3);

% Store trigonometric operations
s_phi = sin(phi_rad);
c_phi = cos(phi_rad);
s_theta = sin(theta_rad);
c_theta = cos(theta_rad);
s_psi = sin(psi_rad);
c_psi = cos(psi_rad);

% Compute NED to body-fixed DCM
C_n2b_11 =  c_theta*c_psi;
C_n2b_21 = -c_phi*s_psi + s_phi*s_theta*c_psi;
C_n2b_31 =  s_phi*s_psi + c_phi*s_theta*c_psi;
C_n2b_12 =  c_theta*s_psi;
C_n2b_22 =  c_phi*c_psi + s_phi*s_theta*s_psi;
C_n2b_32 = -s_phi*c_psi + c_phi*s_theta*s_psi;
C_n2b_13 = -s_theta;
C_n2b_23 =  s_phi*c_theta;
C_n2b_33 =  c_phi*c_theta;

% Convert velocity
u_b_mps = C_n2b_11*u_n_mps + C_n2b_12*v_n_mps + C_n2b_13*w_n_mps;
v_b_mps = C_n2b_21*u_n_mps + C_n2b_22*v_n_mps + C_n2b_23*w_n_mps;
w_b_mps = C_n2b_31*u_n_mps + C_n2b_32*v_n_mps + C_n2b_33*w_n_mps;
vec_b = [u_b_mps v_b_mps w_b_mps]';

== matlab function AirbrakeFlightSim_R2022a/Simulate Sensors/Noisy Sensors/Accelerometer/MATLAB Function ==
  data: astar output; x input; xdot input; r_b_sensor input; gz_n_mps2 input
function astar = simulateIdealAccelerometer(x,xdot,r_b_sensor, gz_n_mps2)
% function astar = simulateAccelerometer(x,xdot,r_sensor)
% Generates idealized accelerometer readings
%
% Inputs:
%   x - state vector [u v w p q r phi theta psi p_N p_E p_D]'
%   xdot - state derivative
%   r_sensor - position vector of accelerometer w.r.t. vehicle CM
%
% Outputs:
%   astar = idealized accelerometer readings (no bias, drift, noise).
%

% Extract state variables
phi_rad = x(7);  % Euler-angles roll,pitch
theta_rad = x(8);

% Store trigonometric operations
s_phi = sin(phi_rad);
c_phi = cos(phi_rad);
s_theta = sin(theta_rad);
c_theta = cos(theta_rad);

% Define NED to body-fixed rotation 
C_n2b_13 = -s_theta;
C_n2b_23 = s_phi*c_theta;
C_n2b_33 = c_phi*c_theta;

% Resolve gravity in body-fixed
gx_b_mps2 = C_n2b_13*gz_n_mps2;
gy_b_mps2 = C_n2b_23*gz_n_mps2;
gz_b_mps2 = C_n2b_33*gz_n_mps2;
g_b_mps2 = [gx_b_mps2 gy_b_mps2 gz_b_mps2]';

% Extract vectors
vvec = [x(1) x(2) x(3)]';
vvecdot = [xdot(1) xdot(2) xdot(3)]';
omega = [x(4) x(5) x(6)]';
omegadot = [xdot(4) xdot(5) xdot(6)]';

% Compute idealized accelerometer readings
astar = vvecdot + cross(omega,vvec) + cross(omegadot,r_b_sensor)...
    + cross(omega, cross(omega, r_b_sensor)) - g_b_mps2;
